simulink model "quad_modified_pid"  (Simulink 7.8)
settings: Solver=ode45  StartTime=0.0  StopTime=20  RelTol=1e-3
InitFcn:
  | % load parameters of the default quadrotor
  | disp('Quadrotor parameters loaded by InitFcn')
  | mdl_quadcopter
undefined symbols (not defined in the file or in its folder): quad
libraries: dsparch4 x3, commnoisgen2 x1, simulink x1
settings Model: Creator=deep  LastModifiedBy=siddh_000

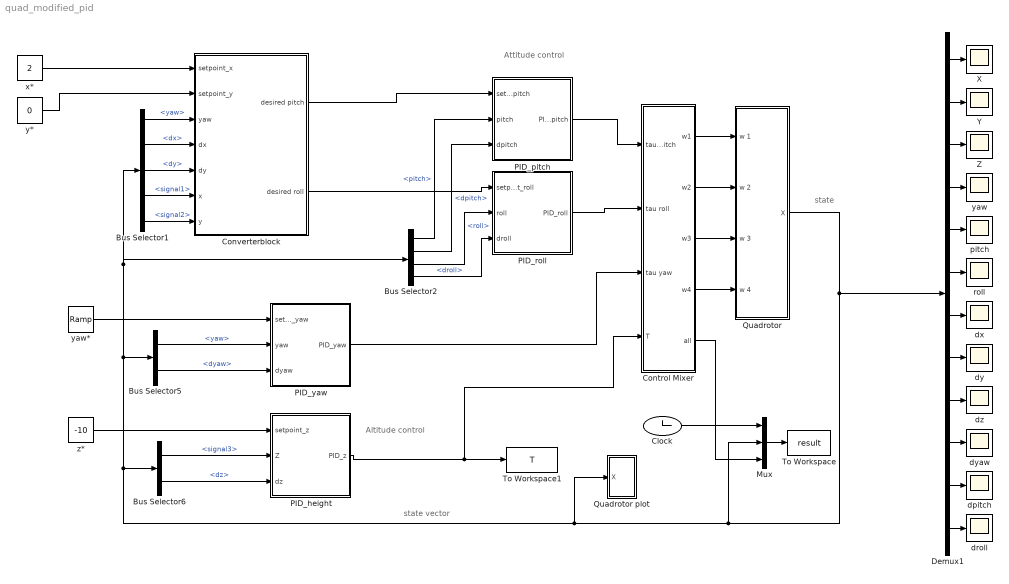
== system quad_modified_pid ==
  note: state vector
  note: state
  note: Attitude control
  note: Altitude control
  Bus Selector1 : BusSelector  OutputSignals=yaw,dx,dy,signal1,signal2
  Bus Selector2 : BusSelector  OutputSignals=pitch,dpitch,roll,droll
  Bus Selector5 : BusSelector  OutputSignals=yaw,dyaw
  Bus Selector6 : BusSelector  OutputSignals=signal3,dz
  Clock : Clock
  Control Mixer : Subsystem  AncestorBlock=roblocks/Dynamics/Control Mixer
  Converterblock : Subsystem  AncestorBlock=roblocks/Dynamics/Control Mixer
  Demux1 : Demux  Outputs=12  BusSelectionMode=on
  Mux : Mux  Inputs=3
  PID_height : Subsystem  AncestorBlock=roblocks/Dynamics/Control Mixer
  PID_pitch : Subsystem  AncestorBlock=roblocks/Dynamics/Control Mixer
  PID_roll : Subsystem  AncestorBlock=roblocks/Dynamics/Control Mixer
  PID_yaw : Subsystem  AncestorBlock=roblocks/Dynamics/Control Mixer
  Quadrotor : Subsystem  AncestorBlock=roblocks/Dynamics/Quadrotor
  Quadrotor plot : Subsystem  AncestorBlock=roblocks/Robot Graphics/Quadrotor plot
  To Workspace : ToWorkspace  VariableName=result  SampleTime=-1  SaveFormat=Array
  To Workspace1 : ToWorkspace  VariableName=T  SampleTime=-1  SaveFormat=Array
  X : Scope
      settings: YMin=-0.04  YMax=0.045
  Y : Scope
      settings: YMin=-0.04  YMax=0.045  SaveName=ScopeData2
  Z : Scope
      settings: YMin=-0.04  YMax=0.045  SaveName=ScopeData3
  dpitch : Scope
      settings: YMin=-0.04  YMax=0.045  SaveName=ScopeData11
  droll : Scope
      settings: YMin=-0.04  YMax=0.045  SaveName=ScopeData12
  dx : Scope
      settings: YMin=-0.04  YMax=0.045  SaveName=ScopeData7
  dy : Scope
      settings: YMin=-0.04  YMax=0.045  SaveName=ScopeData8
  dyaw : Scope
      settings: YMin=-0.04  YMax=0.045  SaveName=ScopeData10
  dz : Scope
      settings: YMin=-0.04  YMax=0.045  SaveName=ScopeData9
  pitch : Scope
      settings: YMin=-0.04  YMax=0.045  SaveName=ScopeData5
  roll : Scope
      settings: YMin=-0.04  YMax=0.045  SaveName=ScopeData6
  x* : Constant  Value=2
  y* : Constant  Value=0
  yaw : Scope
      settings: YMin=-0.04  YMax=0.045  SaveName=ScopeData4
  yaw* : simulink/Sources/Ramp  slope=0  start=0  X0=0
  z* : Constant  Value=-10  SampleTime=0
  wires:
  Control Mixer/1(w1) -> Quadrotor/1(w 1)
  Control Mixer/4(w4) -> Quadrotor/4(w 4)
  Quadrotor/1(X) -> Bus Selector6/1, Bus Selector5/1, Bus Selector1/1, Bus Selector2/1, Quadrotor plot/1(X), Mux/2, Demux1/1
  PID_yaw/1(PID_yaw) -> Control Mixer/3(tau yaw)
  Bus Selector5/1 -> PID_yaw/2(yaw)  "<yaw>"
  z*/1 -> PID_height/1(setpoint_z)
  Mux/1 -> To Workspace/1
  Clock/1 -> Mux/1
  Control Mixer/5(all) -> Mux/3
  Control Mixer/3(w3) -> Quadrotor/3(w 3)
  Control Mixer/2(w2) -> Quadrotor/2(w 2)
  Demux1/1 -> X/1
  Demux1/2 -> Y/1
  Demux1/3 -> Z/1
  Demux1/4 -> yaw/1
  Demux1/5 -> pitch/1
  Demux1/6 -> roll/1
  Demux1/7 -> dx/1
  Demux1/8 -> dy/1
  Demux1/9 -> dz/1
  Demux1/10 -> dyaw/1
  Demux1/11 -> dpitch/1
  Demux1/12 -> droll/1
  Bus Selector6/1 -> PID_height/2(Z)  "<signal3>"
  Bus Selector6/2 -> PID_height/3(dz)  "<dz>"
  PID_height/1(PID_z) -> Control Mixer/4(T), To Workspace1/1
  yaw*/1 -> PID_yaw/1(setpoint_yaw)
  Bus Selector5/2 -> PID_yaw/3(dyaw)  "<dyaw>"
  x*/1 -> Converterblock/1(setpoint_x)
  y*/1 -> Converterblock/2(setpoint_y)
  Bus Selector1/2 -> Converterblock/4(dx)  "<dx>"
  Bus Selector1/1 -> Converterblock/3(yaw)  "<yaw>"
  Bus Selector1/3 -> Converterblock/5(dy)  "<dy>"
  Bus Selector1/4 -> Converterblock/6(x)  "<signal1>"
  Bus Selector1/5 -> Converterblock/7(y)  "<signal2>"
  PID_pitch/1(PID_pitch) -> Control Mixer/1(tau pitch)
  PID_roll/1(PID_roll) -> Control Mixer/2(tau roll)
  Converterblock/1(desired pitch) -> PID_pitch/1(setpoint_pitch)
  Converterblock/2(desired roll) -> PID_roll/1(setpoint_roll)
  Bus Selector2/1 -> PID_pitch/2(pitch)  "<pitch>"
  Bus Selector2/2 -> PID_pitch/3(dpitch)  "<dpitch>"
  Bus Selector2/3 -> PID_roll/2(roll)  "<roll>"
  Bus Selector2/4 -> PID_roll/3(droll)  "<droll>"

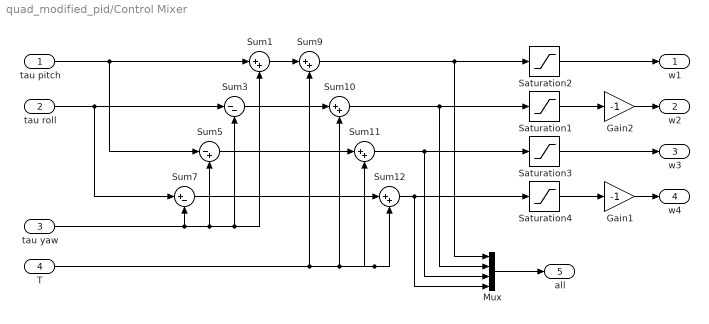
== system quad_modified_pid/Control Mixer ==
  tau pitch : Inport
  tau roll : Inport  Port=2
  tau yaw : Inport  Port=3
  T : Inport  Port=4
  Gain1 : Gain  Gain=-1
  Gain2 : Gain  Gain=-1
  Mux : Mux
  Saturation{1..4} (4 alike) : Saturate  UpperLimit=1000  LowerLimit=700
  Sum{1,9..12} (5 alike) : Sum  Inputs=|++  SaturateOnIntegerOverflow=on  InputSameDT=on  OutDataTypeStr=Inherit: Same as first input
  Sum3 : Sum  Inputs=|--  SaturateOnIntegerOverflow=on  InputSameDT=on  OutDataTypeStr=Inherit: Same as first input
  Sum5 : Sum  Inputs=|-+  SaturateOnIntegerOverflow=on  InputSameDT=on  OutDataTypeStr=Inherit: Same as first input
  Sum7 : Sum  Inputs=|+-  SaturateOnIntegerOverflow=on  InputSameDT=on  OutDataTypeStr=Inherit: Same as first input
  w1 : Outport
  w2 : Outport  Port=2
  w3 : Outport  Port=3
  w4 : Outport  Port=4
  all : Outport  Port=5
  wires:
  tau yaw/1 -> Sum7/2, Sum5/2, Sum3/2, Sum1/2
  Saturation2/1 -> w1/1
  Saturation1/1 -> Gain2/1
  Saturation3/1 -> w3/1
  Saturation4/1 -> Gain1/1
  tau pitch/1 -> Sum1/1, Sum5/1
  Sum1/1 -> Sum9/1
  Sum3/1 -> Sum10/1
  Sum5/1 -> Sum11/1
  Sum7/1 -> Sum12/1
  Sum9/1 -> Mux/1, Saturation2/1
  Sum10/1 -> Saturation1/1, Mux/2
  Sum11/1 -> Saturation3/1, Mux/3
  Sum12/1 -> Saturation4/1, Mux/4
  T/1 -> Sum12/2, Sum11/2, Sum10/2, Sum9/2
  tau roll/1 -> Sum3/1, Sum7/1
  Mux/1 -> all/1
  Gain2/1 -> w2/1
  Gain1/1 -> w4/1

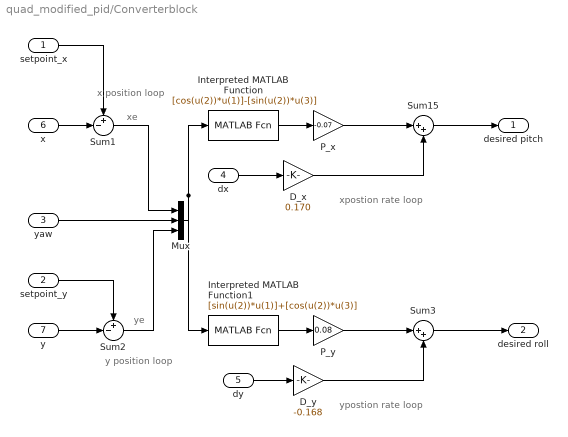
== system quad_modified_pid/Converterblock ==
  note: xpostion rate
      | loop
  note: x position
      | loop
  note: xe
  note: ye
  note: ypostion rate
      | loop
  note: y position loop
  setpoint_x : Inport
  setpoint_y : Inport  Port=2
  yaw : Inport  Port=3
  dx : Inport  Port=4
  dy : Inport  Port=5
  x : Inport  Port=6
  y : Inport  Port=7
  D_x : Gain  Gain=0.170
  D_y : Gain  Gain=-0.168
  Interpreted MATLAB Function : MATLABFcn  MATLABFcn=[cos(u(2))*u(1)]-[sin(u(2))*u(3)]
  Interpreted MATLAB Function1 : MATLABFcn  MATLABFcn=[sin(u(2))*u(1)]+[cos(u(2))*u(3)]
  Mux : Mux  Inputs=3
  P_x : Gain  Gain=-0.07
  P_y : Gain  Gain=0.08
  Sum1 : Sum  Inputs=+-|
  Sum15 : Sum  Inputs=|++
  Sum2 : Sum  Inputs=+-|
  Sum3 : Sum  Inputs=|++
  desired pitch : Outport
  desired roll : Outport  Port=2
  wires:
  setpoint_x/1 -> Sum1/1
  P_x/1 -> Sum15/1
  D_x/1 -> Sum15/2
  Sum15/1 -> desired pitch/1
  x/1 -> Sum1/2
  setpoint_y/1 -> Sum2/1
  y/1 -> Sum2/2
  yaw/1 -> Mux/2
  Sum1/1 -> Mux/1
  Sum2/1 -> Mux/3
  Mux/1 -> Interpreted MATLAB Function/1, Interpreted MATLAB Function1/1
  dx/1 -> D_x/1
  Interpreted MATLAB Function/1 -> P_x/1
  P_y/1 -> Sum3/1
  D_y/1 -> Sum3/2
  Sum3/1 -> desired roll/1
  dy/1 -> D_y/1
  Interpreted MATLAB Function1/1 -> P_y/1

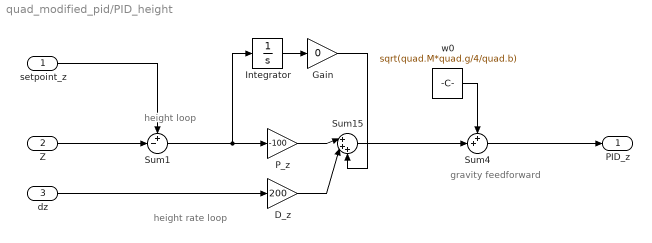
== system quad_modified_pid/PID_height ==
  note: height rate
      | loop
  note: height
      | loop
  note: gravity feedforward
  setpoint_z : Inport
  Z : Inport  Port=2
  dz : Inport  Port=3
  D_z : Gain  Gain=200
  Gain : Gain  Gain=0
  Integrator : Integrator
  P_z : Gain  Gain=-100
  Sum1 : Sum  Inputs=+-|
  Sum15 : Sum  Inputs=|+++
  Sum4 : Sum  Inputs=++|
  w0 : Constant  Value=sqrt(quad.M*quad.g/4/quad.b)  SampleTime=0
  PID_z : Outport
  wires:
  setpoint_z/1 -> Sum1/1
  Sum1/1 -> P_z/1, Integrator/1
  dz/1 -> D_z/1
  P_z/1 -> Sum15/1
  D_z/1 -> Sum15/2
  w0/1 -> Sum4/1
  Sum15/1 -> Sum4/2
  Sum4/1 -> PID_z/1
  Z/1 -> Sum1/2
  Integrator/1 -> Gain/1
  Gain/1 -> Sum15/3

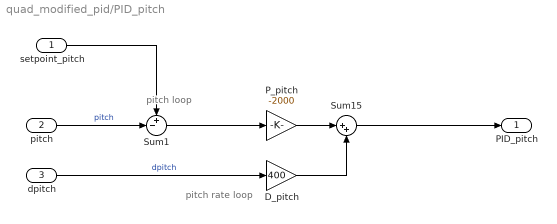
== system quad_modified_pid/PID_pitch ==
  note: pitch rate
      | loop
  note: pitch
      | loop
  setpoint_pitch : Inport
  pitch : Inport  Port=2
  dpitch : Inport  Port=3
  D_pitch : Gain  Gain=400
  P_pitch : Gain  Gain=-2000
  Sum1 : Sum  Inputs=+-|
  Sum15 : Sum  Inputs=|++
  PID_pitch : Outport
  wires:
  setpoint_pitch/1 -> Sum1/1
  pitch/1 -> Sum1/2  "pitch"
  Sum1/1 -> P_pitch/1
  dpitch/1 -> D_pitch/1  "dpitch"
  P_pitch/1 -> Sum15/1
  D_pitch/1 -> Sum15/2
  Sum15/1 -> PID_pitch/1

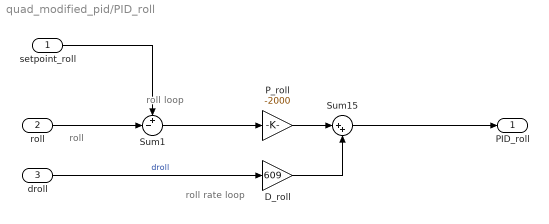
== system quad_modified_pid/PID_roll ==
  note: roll rate
      | loop
  note: roll
      | loop
  note: roll
  setpoint_roll : Inport
  roll : Inport  Port=2
  droll : Inport  Port=3
  D_roll : Gain  Gain=609
  P_roll : Gain  Gain=-2000
  Sum1 : Sum  Inputs=+-|
  Sum15 : Sum  Inputs=|++
  PID_roll : Outport
  wires:
  setpoint_roll/1 -> Sum1/1
  roll/1 -> Sum1/2
  Sum1/1 -> P_roll/1
  droll/1 -> D_roll/1  "droll"
  P_roll/1 -> Sum15/1
  D_roll/1 -> Sum15/2
  Sum15/1 -> PID_roll/1

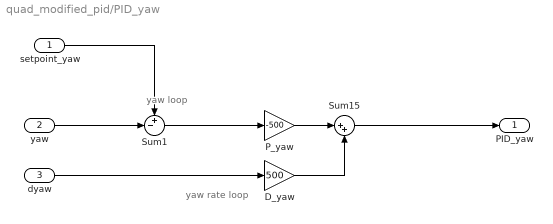
== system quad_modified_pid/PID_yaw ==
  note: yaw rate
      | loop
  note: yaw
      | loop
  setpoint_yaw : Inport
  yaw : Inport  Port=2
  dyaw : Inport  Port=3
  D_yaw : Gain  Gain=500
  P_yaw : Gain  Gain=-500
  Sum1 : Sum  Inputs=+-|
  Sum15 : Sum  Inputs=|++
  PID_yaw : Outport
  wires:
  setpoint_yaw/1 -> Sum1/1
  yaw/1 -> Sum1/2
  Sum1/1 -> P_yaw/1
  dyaw/1 -> D_yaw/1
  P_yaw/1 -> Sum15/1
  D_yaw/1 -> Sum15/2
  Sum15/1 -> PID_yaw/1

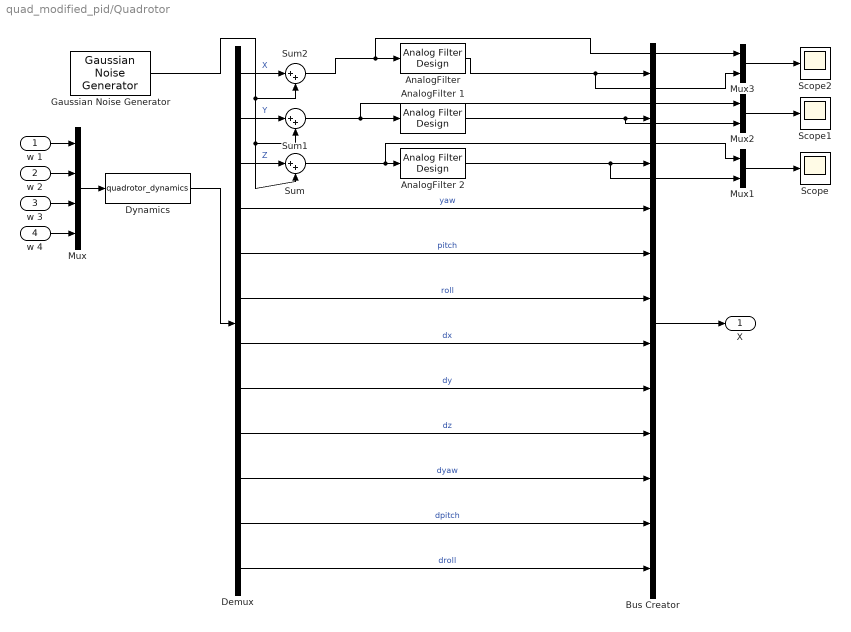
== system quad_modified_pid/Quadrotor ==
  w 1 : Inport
  w 2 : Inport  Port=2
  w 3 : Inport  Port=3
  w 4 : Inport  Port=4
  "AnalogFilter " : dsparch4/Analog Filter Design  method=Butterworth  filttype=Lowpass  N=8  Wlo=10  Whi=80  Rp=2  Rs=40
  "AnalogFilter 1 " : dsparch4/Analog Filter Design  method=Butterworth  filttype=Lowpass  N=8  Wlo=1  Whi=80  Rp=2  Rs=40
  AnalogFilter 2 : dsparch4/Analog Filter Design  method=Butterworth  filttype=Lowpass  N=8  Wlo=10  Whi=80  Rp=2  Rs=40
  Bus Creator : BusCreator  Inputs=12
  Demux : Demux  Outputs=12
  Dynamics : S-Function  FunctionName=quadrotor_dynamics  Parameters=quad  EnableBusSupport=off
  Gaussian Noise Generator : commnoisgen2/Gaussian Noise Generator  m=0  d=0.01  s=0  Ts=0.01  frameBased=off  sampPerFrame=1  orient=off  outDataType=double
  Mux : Mux
  Mux1 : Mux  Inputs=2
  Mux2 : Mux  Inputs=2
  Mux3 : Mux  Inputs=2
  Scope : Scope
  Scope1 : Scope
      settings: SaveName=ScopeData13
  Scope2 : Scope
      settings: YMin=1.7  YMax=2.4  SaveName=ScopeData14
  Sum : Sum  Inputs=|++
  Sum1 : Sum  Inputs=|++
  Sum2 : Sum  Inputs=|++
  X : Outport
  wires:
  Mux/1 -> Dynamics/1
  Demux/4 -> Bus Creator/4  "yaw"
  Demux/5 -> Bus Creator/5  "pitch"
  w 1/1 -> Mux/1
  w 2/1 -> Mux/2
  w 3/1 -> Mux/3
  w 4/1 -> Mux/4
  Demux/7 -> Bus Creator/7  "dx"
  Demux/9 -> Bus Creator/9  "dz"
  Demux/6 -> Bus Creator/6  "roll"
  Demux/8 -> Bus Creator/8  "dy"
  Bus Creator/1 -> X/1
  Dynamics/1 -> Demux/1
  Demux/10 -> Bus Creator/10  "dyaw"
  Demux/11 -> Bus Creator/11  "dpitch"
  Demux/12 -> Bus Creator/12  "droll"
  Demux/3 -> Sum/1  "Z"
  Gaussian Noise Generator/1 -> Sum/2, Sum1/2, Sum2/2
  Sum/1 -> AnalogFilter 2/1, Mux1/1
  Mux1/1 -> Scope/1
  AnalogFilter 2/1 -> Bus Creator/3, Mux1/2
  Demux/2 -> Sum1/1  "Y"
  Sum1/1 -> "AnalogFilter 1 "/1, Mux2/1
  "AnalogFilter 1 "/1 -> Mux2/2, Bus Creator/2
  Demux/1 -> Sum2/1  "X"
  Sum2/1 -> "AnalogFilter "/1, Mux3/1
  "AnalogFilter "/1 -> Bus Creator/1, Mux3/2
  Mux3/1 -> Scope2/1
  Mux2/1 -> Scope1/1

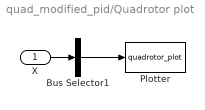
== system quad_modified_pid/Quadrotor plot ==
  X : Inport
  Bus Selector1 : BusSelector  OutputSignals=signal1,signal2,signal3,yaw,pitch,roll  OutputAsBus=on
  Plotter : S-Function  FunctionName=quadrotor_plot  Parameters=[2,10], 1, 1  EnableBusSupport=off
  wires:
  X/1 -> Bus Selector1/1
  Bus Selector1/1 -> Plotter/1
